simulink model "bit8reg"  (R2020a)
settings: Solver=VariableStepAuto  StartTime=0.0  StopTime=10.0  RelTol=1e-3
libraries: simulink_extras x8
settings Model: Creator=kishan  LastModifiedBy=kishan

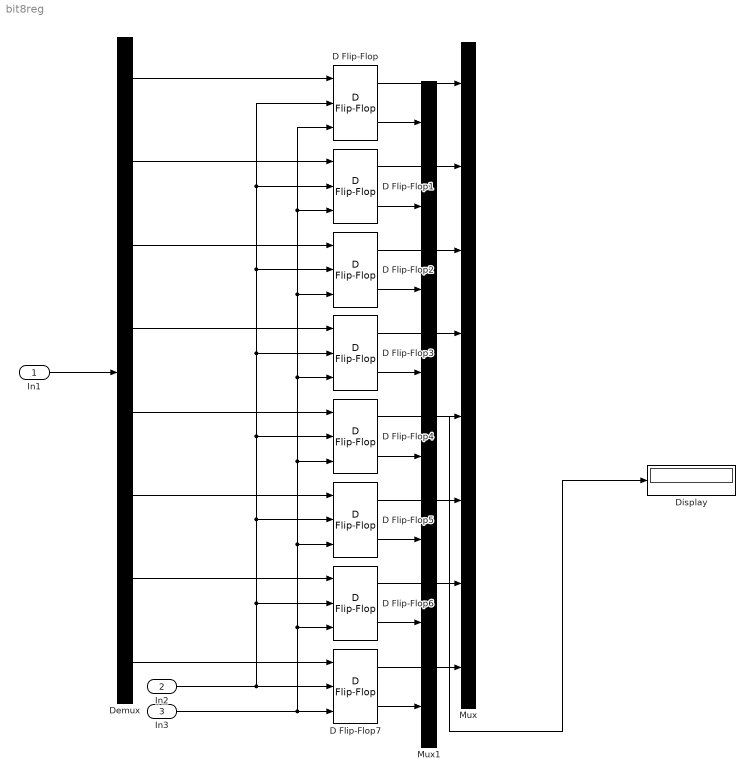
== system bit8reg ==
  In1 : Inport
  In2 : Inport  Port=2
  In3 : Inport  Port=3
  D Flip-Flop{,1..7} (8 alike) : simulink_extras/Flip Flops/D Flip-Flop
  Demux : Demux  Outputs=8
  Display : Display
  Mux : Mux  Inputs=8
  Mux1 : Mux  Inputs=8
  wires:
  In3/1 -> D Flip-Flop7/3, D Flip-Flop6/3, D Flip-Flop5/3, D Flip-Flop4/3, D Flip-Flop3/3, D Flip-Flop2/3, D Flip-Flop1/3, D Flip-Flop/3
  In2/1 -> D Flip-Flop7/2, D Flip-Flop6/2, D Flip-Flop5/2, D Flip-Flop4/2, D Flip-Flop3/2, D Flip-Flop2/2, D Flip-Flop/2, D Flip-Flop1/2
  Demux/1 -> D Flip-Flop/1
  Demux/2 -> D Flip-Flop1/1
  Demux/3 -> D Flip-Flop2/1
  Demux/4 -> D Flip-Flop3/1
  Demux/5 -> D Flip-Flop4/1
  Demux/6 -> D Flip-Flop5/1
  Demux/7 -> D Flip-Flop6/1
  Demux/8 -> D Flip-Flop7/1
  In1/1 -> Demux/1
  D Flip-Flop/1 -> Mux/1
  D Flip-Flop1/1 -> Mux/2
  D Flip-Flop2/1 -> Mux/3
  D Flip-Flop3/1 -> Mux/4
  D Flip-Flop4/1 -> Mux/5
  D Flip-Flop5/1 -> Mux/6
  D Flip-Flop6/1 -> Mux/7
  D Flip-Flop7/1 -> Mux/8
  D Flip-Flop/2 -> Mux1/1
  D Flip-Flop1/2 -> Mux1/2
  D Flip-Flop2/2 -> Mux1/3
  D Flip-Flop3/2 -> Mux1/4
  D Flip-Flop4/2 -> Mux1/5
  D Flip-Flop5/2 -> Mux1/6
  D Flip-Flop6/2 -> Mux1/7
  D Flip-Flop7/2 -> Mux1/8
  Mux1/1 -> Display/1
